simulink model "SampleApplication"  (R2024b)
settings: Solver=VariableStepAuto  StartTime=0.0  StopTime=100  RelTol=1e-3
libraries: slrealtimeutilitieslib x5, slrealtimeiplib x3, etargetslib x2
settings Model: Creator=mergurtu  LastModifiedBy=saijaz
settings OptimizationCC: UseDivisionForNetSlopeComputation=on
settings RTWCC: GPUComputeCapability=3.5

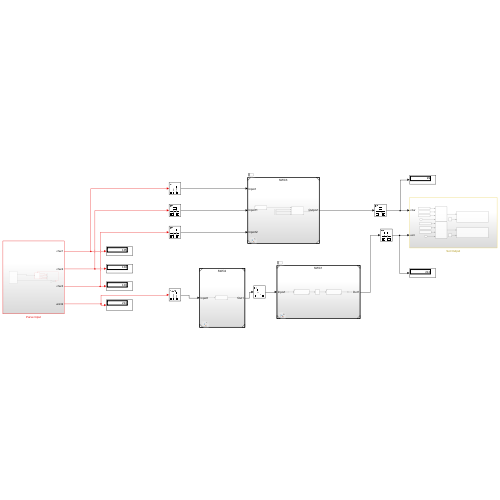
[thumbnail: Simulink's stored preview of the top-level diagram]
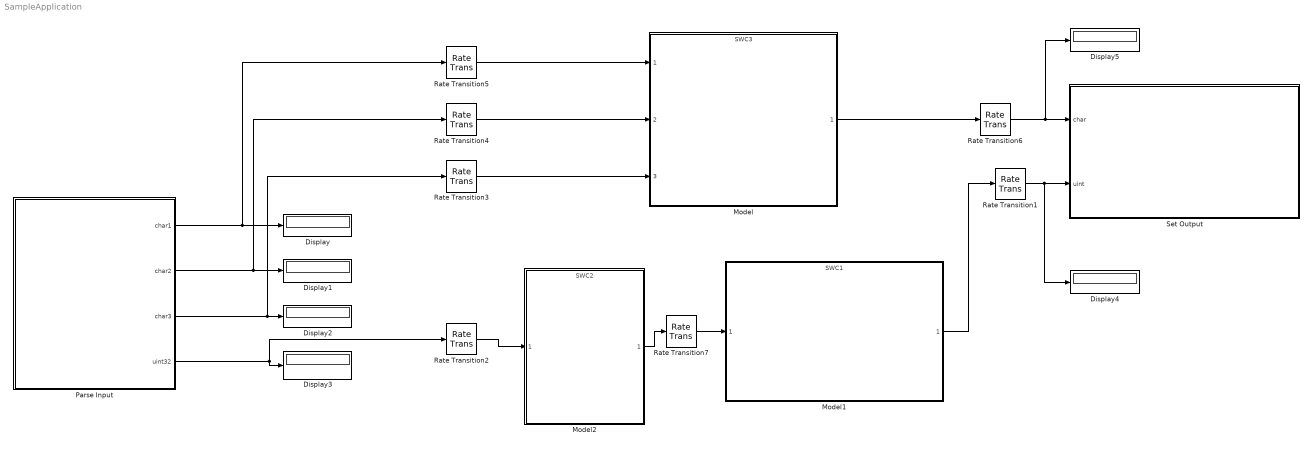
== system SampleApplication ==
  Display{,1..5} (6 alike) : Display
  Model : ModelReference  ModelNameDialog=SWC3.slx  SimulationMode=Normal  ScheduleRates=on  ScheduleRatesWith=Schedule Editor  ModelReferenceVersion=1.11
  Model1 : ModelReference  ModelNameDialog=SWC1.slx  SimulationMode=Normal  ScheduleRates=on  ScheduleRatesWith=Schedule Editor  ModelReferenceVersion=4.0
  Model2 : ModelReference  ModelNameDialog=SWC2.slx  SimulationMode=Normal  ModelReferenceVersion=4.0
  Parse Input : Subsystem
  Rate Transition{1..7} (7 alike) : RateTransition
  Set Output : Subsystem
  wires:
  Parse Input/2(char2) -> Rate Transition4/1, Display1/1
  Parse Input/1(char1) -> Rate Transition5/1, Display/1
  Parse Input/4(uint32) -> Rate Transition2/1, Display3/1
  Parse Input/3(char3) -> Rate Transition3/1, Display2/1
  Model1/1 -> Rate Transition1/1
  Model/1 -> Rate Transition6/1
  Rate Transition1/1 -> Display4/1, Set Output/2(uint)
  Rate Transition2/1 -> Model2/1
  Rate Transition3/1 -> Model/3
  Rate Transition4/1 -> Model/2
  Rate Transition5/1 -> Model/1
  Rate Transition6/1 -> Display5/1, Set Output/1(char)
  Model2/1 -> Rate Transition7/1
  Rate Transition7/1 -> Model1/1

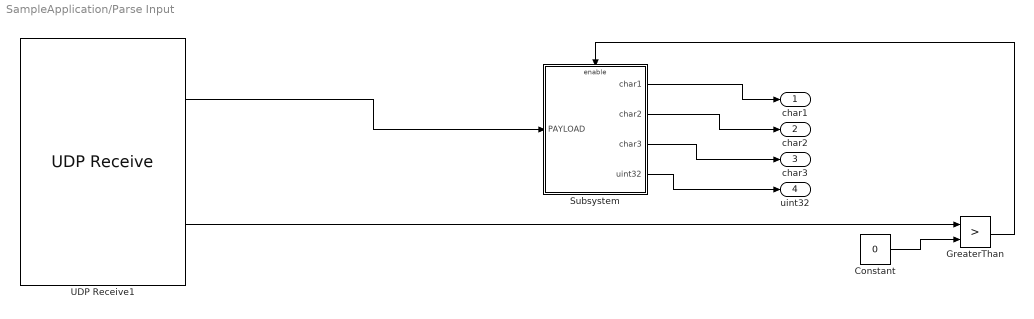
== system SampleApplication/Parse Input ==
  Constant : Constant  Value=0
  GreaterThan : RelationalOperator  Operator=>  OutDataTypeStr=boolean  RndMeth=Simplest  InputSameDT=off
  Subsystem : Subsystem
  UDP Receive1 : slrealtimeiplib/UDP Receive  useHostTargetConn=off  ipAddress=10.42.0.10  localPort=5002  rcvWidth=20  rcvFmAny=on  fmAddress='10.10.10.10'  sampleTime=-1  enableMessage=off  maxPackets=1
  char1 : Outport
  char2 : Outport  Port=2
  char3 : Outport  Port=3
  uint32 : Outport  Port=4
  wires:
  GreaterThan/1 -> Subsystem/Enable
  Constant/1 -> GreaterThan/2
  Subsystem/1(char1) -> char1/1
  Subsystem/2(char2) -> char2/1
  Subsystem/3(char3) -> char3/1
  Subsystem/4(uint32) -> uint32/1
  UDP Receive1/2 -> GreaterThan/1
  UDP Receive1/1 -> Subsystem/1(PAYLOAD)

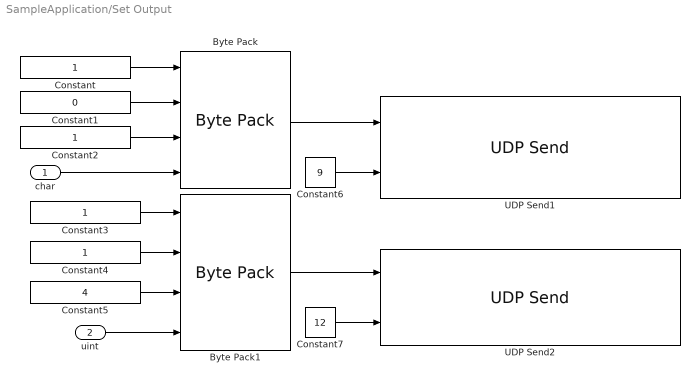
== system SampleApplication/Set Output ==
  char : Inport
  uint : Inport  Port=2
  Byte Pack : etargetslib/Byte Pack  datatypes={'uint16','uint16','uint32','uint8'}  byteAlign=1
  Byte Pack1 : etargetslib/Byte Pack  datatypes={'uint16','uint16','uint32','uint32'}  byteAlign=1
  Constant : Constant  OutDataTypeStr=uint16
  Constant1 : Constant  Value=0  OutDataTypeStr=uint16
  Constant2 : Constant  OutDataTypeStr=uint32
  Constant3 : Constant  OutDataTypeStr=uint16
  Constant4 : Constant  OutDataTypeStr=uint16
  Constant5 : Constant  Value=4  OutDataTypeStr=uint32
  Constant6 : Constant  Value=9
  Constant7 : Constant  Value=12
  UDP Send1 : slrealtimeiplib/UDP Send  useHostTargetConn=off  toAddress='10.42.0.11'  toPort=5001  sampleTime=0.1  enableMessage=off
  UDP Send2 : slrealtimeiplib/UDP Send  useHostTargetConn=off  toAddress='10.42.0.11'  toPort=5001  sampleTime=0.05  enableMessage=off
  wires:
  char/1 -> Byte Pack/4
  Constant/1 -> Byte Pack/1
  Constant1/1 -> Byte Pack/2
  Constant2/1 -> Byte Pack/3
  Constant3/1 -> Byte Pack1/1
  Constant4/1 -> Byte Pack1/2
  Constant5/1 -> Byte Pack1/3
  uint/1 -> Byte Pack1/4
  Byte Pack1/1 -> UDP Send2/1
  Byte Pack/1 -> UDP Send1/1
  Constant6/1 -> UDP Send1/2
  Constant7/1 -> UDP Send2/2

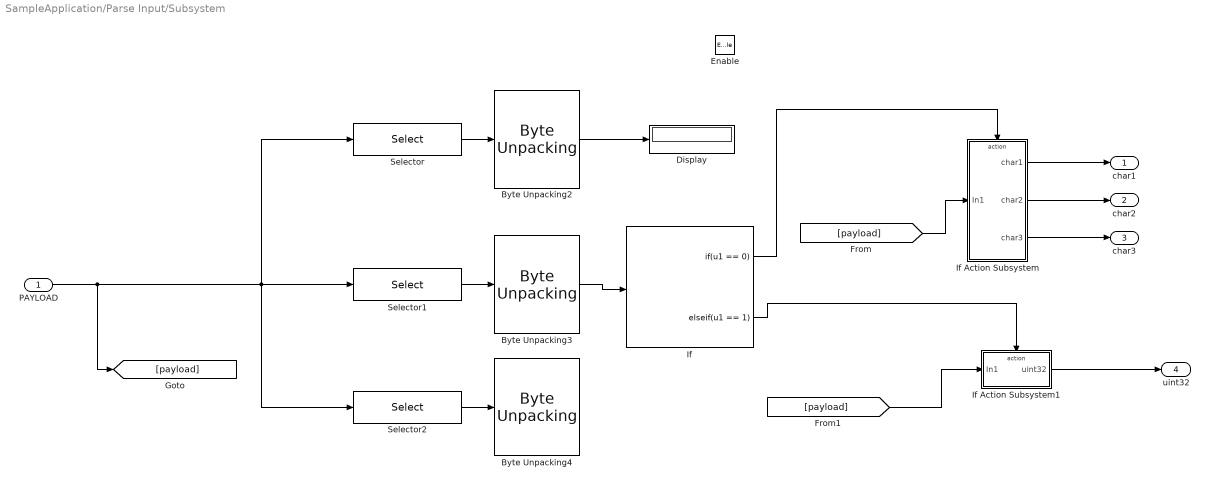
== system SampleApplication/Parse Input/Subsystem ==
  PAYLOAD : Inport
  Enable : EnablePort
  Byte Unpacking2 : slrealtimeutilitieslib/Byte Unpacking  MaskUnpackedDataTypes={'uint16'}  MaskUnpackedDataSizes={[1]}  MaskAlignment=1
  Byte Unpacking3 : slrealtimeutilitieslib/Byte Unpacking  MaskUnpackedDataTypes={'uint16'}  MaskUnpackedDataSizes={[1]}  MaskAlignment=1
  Byte Unpacking4 : slrealtimeutilitieslib/Byte Unpacking  MaskUnpackedDataTypes={'uint32'}  MaskUnpackedDataSizes={[1]}  MaskAlignment=1
  Display : Display
  If : If  IfExpression=u1 == 0  ElseIfExpressions=u1 == 1  ShowElse=off
  If Action Subsystem : Subsystem  TreatAsAtomicUnit=on
  If Action Subsystem1 : Subsystem  TreatAsAtomicUnit=on
  Selector : Selector  InputPortWidth=20  IndexOptions=Index vector (dialog)  Indices=[1,2]  OutputSizes=1
  Selector1 : Selector  InputPortWidth=20  IndexOptions=Index vector (dialog)  Indices=[3,4]  OutputSizes=1
  Selector2 : Selector  InputPortWidth=20  IndexOptions=Index vector (dialog)  Indices=[5,6,7,8]  OutputSizes=1
  char1 : Outport
  char2 : Outport  Port=2
  char3 : Outport  Port=3
  uint32 : Outport  Port=4
  wires:
  PAYLOAD/1 -> [payload], Selector/1, Selector2/1, Selector1/1
  Selector/1 -> Byte Unpacking2/1
  Selector2/1 -> Byte Unpacking4/1
  Selector1/1 -> Byte Unpacking3/1
  Byte Unpacking2/1 -> Display/1
  If/1 -> If Action Subsystem/Action
  If/2 -> If Action Subsystem1/Action
  Byte Unpacking3/1 -> If/1
  [payload] -> If Action Subsystem/1(In1)
  [payload] -> If Action Subsystem1/1(In1)
  If Action Subsystem1/1(uint32) -> uint32/1
  If Action Subsystem/2(char2) -> char2/1
  If Action Subsystem/3(char3) -> char3/1
  If Action Subsystem/1(char1) -> char1/1

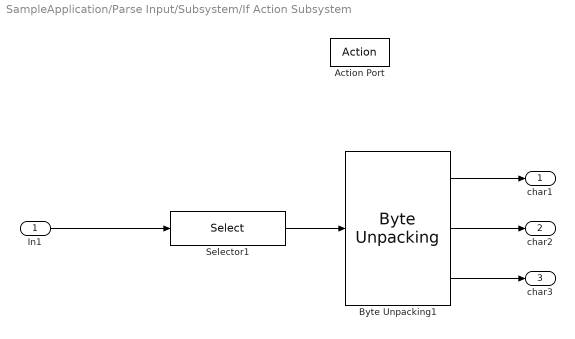
== system SampleApplication/Parse Input/Subsystem/If Action Subsystem ==
  In1 : Inport
  Action Port : ActionPort  ActionPortLabel=if(u1 == 0)
  Byte Unpacking1 : slrealtimeutilitieslib/Byte Unpacking  MaskUnpackedDataTypes={'uint8','uint8','uint8'}  MaskUnpackedDataSizes={[1],[1],[1]}  MaskAlignment=1
  Selector1 : Selector  InputPortWidth=20  IndexOptions=Index vector (dialog)  Indices=[9,10,11]  OutputSizes=1
  char1 : Outport
  char2 : Outport  Port=2
  char3 : Outport  Port=3
  wires:
  Selector1/1 -> Byte Unpacking1/1
  In1/1 -> Selector1/1
  Byte Unpacking1/3 -> char3/1
  Byte Unpacking1/2 -> char2/1
  Byte Unpacking1/1 -> char1/1

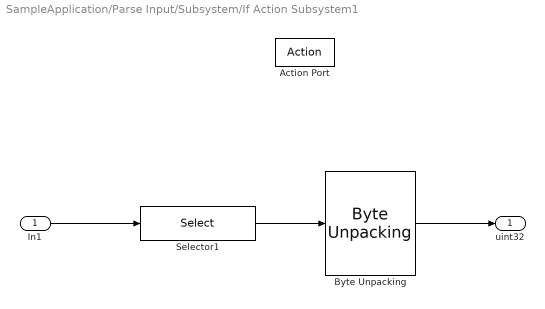
== system SampleApplication/Parse Input/Subsystem/If Action Subsystem1 ==
  In1 : Inport
  Action Port : ActionPort  ActionPortLabel=elseif(u1 == 1)
  Byte Unpacking : slrealtimeutilitieslib/Byte Unpacking  MaskUnpackedDataTypes={'uint32'}  MaskUnpackedDataSizes={[1]}  MaskAlignment=1
  Selector1 : Selector  InputPortWidth=20  IndexOptions=Index vector (dialog)  Indices=[9,10,11,12]  OutputSizes=1
  uint32 : Outport
  wires:
  In1/1 -> Selector1/1
  Selector1/1 -> Byte Unpacking/1
  Byte Unpacking/1 -> uint32/1
